simulink model "DC_motor_simulation"  (R2016a)
settings: Solver=ode45  StartTime=0.0  StopTime=1  RelTol=1e-3
values from neighbouring files (symbols this model uses):
  N = 500    [example1_5.m]    (also in example2_10.m = 20; example2_11.m = 0.00625; ffttest.m = 42)
libraries: powerlib x3, fl_lib x1
settings Model: Creator=zhanghankui  LastModifiedBy=zhanghankui

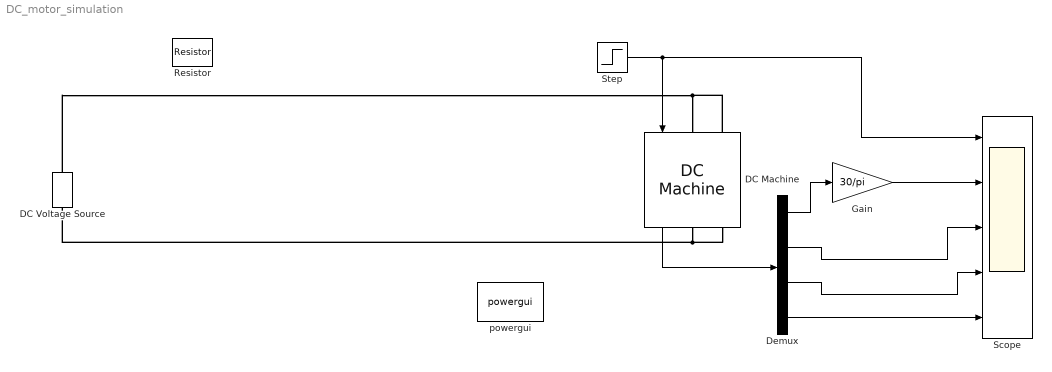
== system DC_motor_simulation ==
  DC Machine : powerlib/Machines/DC Machine  PresetModel=No  MechanicalLoad=Torque TL  FieldType=Wound  ShowDetailedParameters=on  MeasurementBus=off  RLa="[ 0.087  0.0032]"  RLf="[ 181.5  0]"  Laf=0.56  MachineConstant=Torque constant (N.m/A)  Ke=1.8  Kt=1.8  J=0.76  Bm=0  Tf=0  w0=0  Ifinit=0  TsPowergui=0  TsBlock=-1
  DC Voltage Source : powerlib/Electrical Sources/DC Voltage Source  Amplitude=220  Measurements=Voltage
  Demux : Demux
  Gain : Gain  Gain=30/pi
  Resistor : fl_lib/Electrical/Electrical Elements/Resistor  R=1 Ohm  i_specify=off  i_priority=None  i=0 A  v_specify=off  v_priority=None  v=0 V
  Scope : Scope  NumInputPorts=5
  Step : Step  Time=0.5  After=60  SampleTime=0
  powergui : powerlib/powergui  Priority=1  SimulationMode=Continuous  SolverType=Tustin/Backward Euler (TBE)  SampleTime=50e-6  frequency=60  SPID=off  DisableSnubberDevices=off  DisableRonSwitches=off  DisableVfSwitches=off  SwTol=0  DisplayEquations=off  Interpol=off  ExternalGateDelay=off  methode=off  Ts=10  FunctionMessages=off  echomessages=off  HookPort=off  EnableUseOfTLC=off  x0status=blocks  frequencyindice=0  Pbase=100e6  ErrMax=1e-4  Iterations=50  UnitsV=kV  UnitsW=MW  buscounter=0  RestoreLinks=warning  ResistiveCurrentMeasurement=off  Frange=[0:2:500]  Ylog=off  Xlog=on  ShowGrid=off  save=off  variable=ZData  structure=0  ZoomFFT=off  StartTime=0.0  cycles=1  DisplayStyle=1  fundamental=60  FreqAxis=off  MaxFrequency=1000  frequencyindicesteady=1  RmsSteady=1  display=off
  wires:
  Step/1 -> Scope/1, DC Machine/1
  DC Machine/1 -> Demux/1
  Demux/3 -> Scope/4
  Demux/4 -> Scope/5
  Demux/1 -> Gain/1
  Gain/1 -> Scope/2
  Demux/2 -> Scope/3
  connections:
  DC Voltage Source/RConn1 -- DC Machine/LConn2 -- DC Machine/LConn1
  DC Machine/RConn1 -- DC Voltage Source/LConn1 -- DC Machine/RConn2
